simulink model "QPSK"  (R2015a)
settings: Solver=FixedStepDiscrete  SolverMode=SingleTasking  StartTime=0.0  StopTime=(12+226)*8  RelTol=1e-3
libraries: dspsrcs4 x2, dspsigops x2, dspstat3 x1
settings Model: CovModelRefEnable=off  Creator=coltmt  LastModifiedBy=ecenstudent
settings DataIOCC: SaveFormat=Dataset
settings HardwareCC: ProdBitPerPointer=64  ProdLargestAtomicFloat=Float  ProdIntDivRoundTo=Zero  ProdEndianess=LittleEndian  ProdHWDeviceType=Specified
settings GRTTargetCC: GeneratePreprocessorConditionals=Use local settings

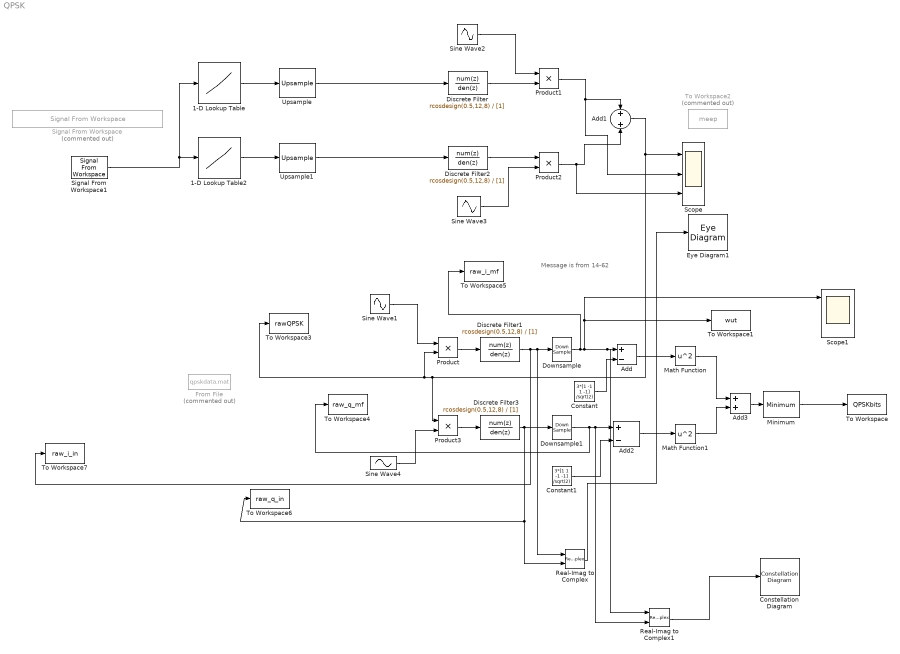
== system QPSK ==
  note: Message is from 14-62
  1-D Lookup Table : Lookup_n-D  NumberOfTableDimensions=1  BreakpointsForDimension1=[0 1 2 3]  Table=[1 -1 1 -1]*3/sqrt(2)  InternalRulePriority=Speed  RndMeth=Simplest  InputSameDT=on
  1-D Lookup Table2 : Lookup_n-D  NumberOfTableDimensions=1  BreakpointsForDimension1=[0 1 2 3]  Table=[1 1 -1 -1]*3/sqrt(2)  InternalRulePriority=Speed  RndMeth=Simplest  InputSameDT=on
  Add : Sum  Inputs=+-
  Add1 : Sum
  Add2 : Sum  Inputs=+-
  Add3 : Sum
  Constant : Constant  Value=3*[1 -1 1 -1] /sqrt(2)
  Constant1 : Constant  Value=3*[1 1 -1 -1] /sqrt(2)
  Constellation Diagram : ConstellationDiagram
  Discrete Filter{,1..3} (4 alike) : DiscreteFilter  Numerator=rcosdesign(0.5,12,8)  Denominator=[1]
  Downsample : DownSample  N=8  InputProcessing=Inherited (this choice will be removed - see release notes)  RateOptions=Allow multirate processing
  Downsample1 : DownSample  N=8  InputProcessing=Inherited (this choice will be removed - see release notes)  RateOptions=Allow multirate processing
  Eye Diagram1 : EyeDiagram
  From File : FromFile  Commented=on  FileName=qpskdata.mat  SampleTime=1
  Math Function : Math  Operator=square  SaturateOnIntegerOverflow=on
  Math Function1 : Math  Operator=square  SaturateOnIntegerOverflow=on
  Minimum : dspstat3/Minimum  fcn=Index  reset=None  InputProcessing=Columns as channels (frame based)  indexBase=Zero  operateOver=Each column  Dimension=1  colComp=off  operation=minimum  roiEnable=off  roiType=Rectangles  roiPortion=Entire ROI  roiOutput=Individual statistics for each ROI  roiFlag=off  roundingMode=Floor  overflowMode=off
  Product{,1..3} (4 alike) : Product
  Real-Imag to Complex : RealImagToComplex
  Real-Imag to Complex1 : RealImagToComplex
  Scope : Scope  NumInputPorts=3
      settings: YMin=-5~-5~-5  YMax=5~5~5
  Scope1 : Scope  NumInputPorts=3
      settings: YMin=-0.60017~-5~-5  YMax=1.16884~5~5
  Signal From Workspace : dspsrcs4/Signal From Workspace  Commented=on  X=[1 2 3 0 0 2 3 1 3 2 1 0 3 2 0 2 0 1 4 2 3 1 0 2 3 1 2 3 0 3 2 1 2 3 0 2 3 3 1 2 3 1 2 3 1 2 3 1 2 1 2 1 2 2 1 2 1 2 1 2 1 2 1 2 1 2 1 2 1 2 1 0 0 3 2 0 1 2 0 1 3 2 3 1 1 1 1 1 0 0 0 1 1 0 0 1 1 1 1 2 1 0 3 0 2 3 3 0 2 3 2 0 0]  Ts=8  nsamps=1  OutputAfterFinalValue=Setting to zero  ignoreOrWarnInputAndFrameLengths=off
  Signal From Workspace1 : dspsrcs4/Signal From Workspace  X=[2,2,3,2,1,3,2,1,0]  Ts=8  nsamps=1  OutputAfterFinalValue=Setting to zero  ignoreOrWarnInputAndFrameLengths=off
  Sine Wave1 : Sin  Amplitude=sqrt(2)  Frequency=2*pi/4  Phase=pi/2  SampleTime=1
  Sine Wave2 : Sin  Amplitude=sqrt(2)  Frequency=2*pi/4  Phase=pi/2  SampleTime=1
  Sine Wave3 : Sin  Amplitude=-sqrt(2)  Frequency=2*pi/4  SampleTime=1
  Sine Wave4 : Sin  Amplitude=-sqrt(2)  Frequency=2*pi/4  SampleTime=1
  To Workspace : ToWorkspace  VariableName=QPSKbits  SampleTime=-1
      settings: Save2DSignal=2-D array (concatenate along first dimension)
  To Workspace1 : ToWorkspace  VariableName=wut  SampleTime=-1
      settings: Save2DSignal=2-D array (concatenate along first dimension)
  To Workspace2 : ToWorkspace  Commented=on  VariableName=meep  SampleTime=-1
      settings: Save2DSignal=2-D array (concatenate along first dimension)
  To Workspace3 : ToWorkspace  VariableName=rawQPSK  SampleTime=-1
      settings: Save2DSignal=2-D array (concatenate along first dimension)
  To Workspace4 : ToWorkspace  VariableName=raw_q_mf  SampleTime=-1
      settings: Save2DSignal=2-D array (concatenate along first dimension)
  To Workspace5 : ToWorkspace  VariableName=raw_i_mf  SampleTime=-1
      settings: Save2DSignal=2-D array (concatenate along first dimension)
  To Workspace6 : ToWorkspace  VariableName=raw_q_in  SampleTime=-1
      settings: Save2DSignal=2-D array (concatenate along first dimension)
  To Workspace7 : ToWorkspace  VariableName=raw_i_in  SampleTime=-1
      settings: Save2DSignal=2-D array (concatenate along first dimension)
  Upsample : dspsigops/Upsample  N=8  phase=0  InputProcessing=Inherited (this choice will be removed - see release notes)  RateOptions=Allow multirate processing  ic=0  mode=Unused parameter value
  Upsample1 : dspsigops/Upsample  N=8  phase=0  InputProcessing=Inherited (this choice will be removed - see release notes)  RateOptions=Allow multirate processing  ic=0  mode=Unused parameter value
  wires:
  1-D Lookup Table/1 -> Upsample/1
  1-D Lookup Table2/1 -> Upsample1/1
  Discrete Filter/1 -> Product1/2
  Sine Wave2/1 -> Product1/1
  Discrete Filter2/1 -> Product2/1
  Sine Wave3/1 -> Product2/2
  Product2/1 -> Scope/3, Add1/2
  Product1/1 -> Scope/2, Add1/1
  Sine Wave1/1 -> Product/1
  Sine Wave4/1 -> Product3/2
  Product/1 -> Discrete Filter1/1
  Product3/1 -> Discrete Filter3/1
  Discrete Filter1/1 -> To Workspace7/1, Real-Imag to Complex/1, Downsample/1
  Discrete Filter3/1 -> To Workspace6/1, Real-Imag to Complex/2, Downsample1/1
  Constant1/1 -> Add2/2
  Constant/1 -> Add/2
  Add/1 -> Math Function/1
  Add2/1 -> Math Function1/1
  Math Function/1 -> Add3/1
  Math Function1/1 -> Add3/2
  Add3/1 -> Minimum/1
  Minimum/1 -> To Workspace/1
  Downsample/1 -> To Workspace5/1, Real-Imag to Complex1/1, Add/1, To Workspace1/1, Scope1/1
  Real-Imag to Complex/1 -> Eye Diagram1/1
  Real-Imag to Complex1/1 -> Constellation Diagram/1
  Add1/1 -> Product3/1, To Workspace3/1, Product/2, Scope/1
  Upsample/1 -> Discrete Filter/1
  Upsample1/1 -> Discrete Filter2/1
  Signal From Workspace1/1 -> 1-D Lookup Table2/1, 1-D Lookup Table/1
  Downsample1/1 -> To Workspace4/1, Real-Imag to Complex1/2, Add2/1
